simulink model "CHM2StateCtrl"  (R2018b)
settings: Solver=FixedStepDiscrete  StartTime=0.0  StopTime=10.0  FixedStep=0.01  RelTol=1e-3
undefined symbols (not defined in the file or in its folder): KeSMSuChmReqDurnTm_Val
settings Model: Creator=sn2xws  LastModifiedBy=sn2xws
settings DataIOCC: SaveFormat=StructureWithTime
settings OptimizationCC: DefaultParameterBehavior=Inlined  EnhancedBackFolding=on  PassReuseOutputArgsAs=Individual arguments  ZeroExternalMemoryAtStartup=off  ZeroInternalMemoryAtStartup=off  OptimizeBlockOrder=speed  DifferentSizesBufferReuse=on  OptimizationCustomize=off
settings DebuggingCC: ParameterTunabilityLossMsg=error
settings ModelReferenceCC: ModelReferenceNumInstancesAllowed=Single
settings SFSimCC: MATLABDynamicMemAlloc=off
settings RTWCC: SystemTargetFile=autosar.tlc  GenCodeOnly=on  TemplateMakefile=ert_default_tmf  Description=AUTOSAR  GenerateReport=on  IncludeHyperlinkInReport=on  LaunchReport=on  GenerateTraceInfo=on  GenerateTraceReport=on  GenerateTraceReportSl=on  GenerateTraceReportSf=on  GenerateTraceReportEml=on  GenerateCodeMetricsReport=on
settings CodeAppCC: ForceParamTrailComments=on  IgnoreCustomStorageClasses=off  OperatorAnnotations=on  SimulinkDataObjDesc=on  SFDataObjDesc=on  InsertBlockDesc=on
settings STFCustomTargetCC: TargetLangStandard=C99 (ISO)  MultiwordLength=256  ParMdlRefBuildCompliant=on  CompOptLevelCompliant=on  IncludeMdlTerminateFcn=off  CombineOutputUpdateFcns=on  SuppressErrorStatus=on  ERTCustomFileBanners=on  SupportNonFinite=off  SupportComplex=off  SupportContinuousTime=off  SupportNonInlinedSFcns=off  RemoveResetFunc=on  MATLABClassNameForMDSCustomization=Simulink.SoftwareTarget.ERTCustomization  AutosarCompliant=on  UseToolchainInfoCompliant=on  LookupTableObjectStructAxisOrder=2,1,3,4,...  LUTObjectStructOrderEvenSpacing=Size,Table,Breakpoints  SystemTargetFile=autosar.tlc
settings ERTTargetCC: TargetLangStandard=C99 (ISO)  ConcurrentExecutionCompliant=off  IncludeMdlTerminateFcn=off  SuppressErrorStatus=on  SupportNonFinite=off  SupportComplex=off  ModelStepFunctionPrototypeControlCompliant=off  CPPClassGenCompliant=off  AutosarCompliant=on  LookupTableObjectStructAxisOrder=2,1,3,4,...  LUTObjectStructOrderEvenSpacing=Size,Table,Breakpoints  InlinedParameterPlacement=NonHierarchical  ERTCustomFileTemplate=example_file_process.tlc  ERTFilePackagingFormat=Compact

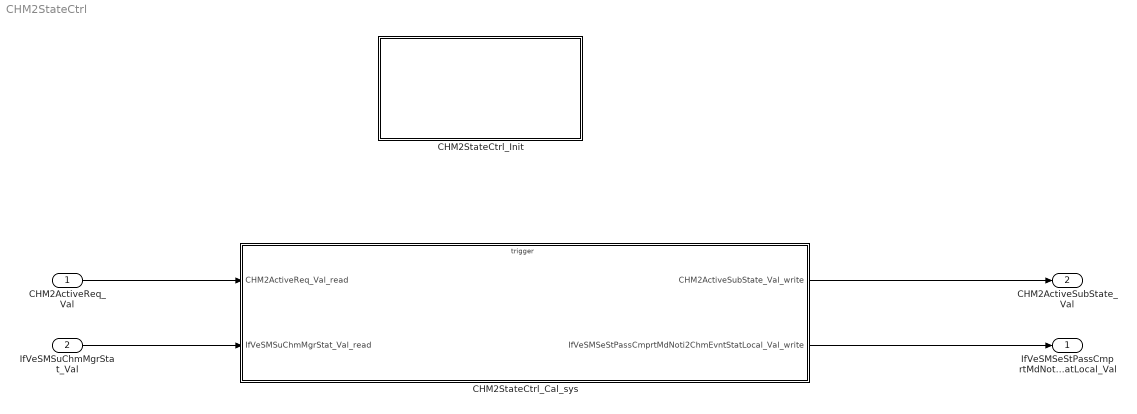
== system CHM2StateCtrl ==
  CHM2ActiveReq_Val : Inport  OutDataTypeStr=boolean  PortDimensions=1
  IfVeSMSuChmMgrStat_Val : Inport  Port=2  OutDataTypeStr=uint16  PortDimensions=1
  CHM2StateCtrl_Cal_sys : Subsystem
  CHM2StateCtrl_Init : Subsystem
  IfVeSMSeStPassCmprtMdNoti2ChmEvntStatLocal_Val : Outport  OutDataTypeStr=Enum: EventSts1  PortDimensions=1
  CHM2ActiveSubState_Val : Outport  Port=2  OutDataTypeStr=boolean  PortDimensions=1
  wires:
  CHM2ActiveReq_Val/1 -> CHM2StateCtrl_Cal_sys/1(CHM2ActiveReq_Val_read)
  IfVeSMSuChmMgrStat_Val/1 -> CHM2StateCtrl_Cal_sys/2(IfVeSMSuChmMgrStat_Val_read)
  CHM2StateCtrl_Cal_sys/1(CHM2ActiveSubState_Val_write) -> CHM2ActiveSubState_Val/1
  CHM2StateCtrl_Cal_sys/2(IfVeSMSeStPassCmprtMdNoti2ChmEvntStatLocal_Val_write) -> IfVeSMSeStPassCmprtMdNoti2ChmEvntStatLocal_Val/1

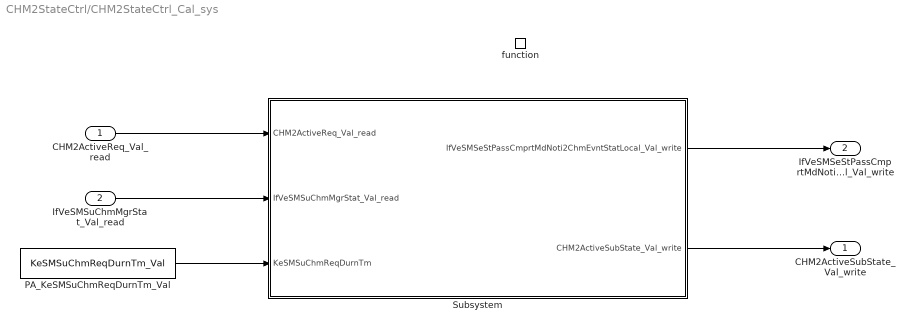
== system CHM2StateCtrl/CHM2StateCtrl_Cal_sys ==
  CHM2ActiveReq_Val_read : Inport
  IfVeSMSuChmMgrStat_Val_read : Inport  Port=2
  function : TriggerPort  TriggerType=function-call  IsSimulinkFunction=on  FunctionName=CHM2StateCtrl_Cal  VariantControl=(inherit)
  PA_KeSMSuChmReqDurnTm_Val : Constant  Value=KeSMSuChmReqDurnTm_Val
  Subsystem : Subsystem
  CHM2ActiveSubState_Val_write : Outport
      settings: EnsureOutportIsVirtual=on
  IfVeSMSeStPassCmprtMdNoti2ChmEvntStatLocal_Val_write : Outport  Port=2
      settings: EnsureOutportIsVirtual=on
  wires:
  Subsystem/2(CHM2ActiveSubState_Val_write) -> CHM2ActiveSubState_Val_write/1
  Subsystem/1(IfVeSMSeStPassCmprtMdNoti2ChmEvntStatLocal_Val_write) -> IfVeSMSeStPassCmprtMdNoti2ChmEvntStatLocal_Val_write/1
  CHM2ActiveReq_Val_read/1 -> Subsystem/1(CHM2ActiveReq_Val_read)
  IfVeSMSuChmMgrStat_Val_read/1 -> Subsystem/2(IfVeSMSuChmMgrStat_Val_read)
  PA_KeSMSuChmReqDurnTm_Val/1 -> Subsystem/3(KeSMSuChmReqDurnTm)

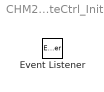
== system CHM2StateCtrl/CHM2StateCtrl_Init ==
  Event Listener : EventListener  EventName=reset

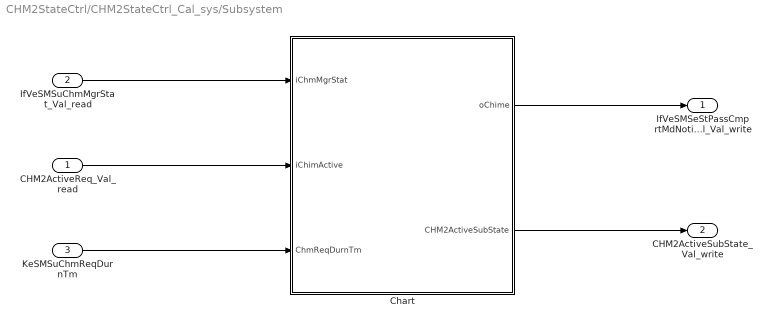
== system CHM2StateCtrl/CHM2StateCtrl_Cal_sys/Subsystem ==
  CHM2ActiveReq_Val_read : Inport
  IfVeSMSuChmMgrStat_Val_read : Inport  Port=2
  KeSMSuChmReqDurnTm : Inport  Port=3
  Chart : Stateflow chart  TreatAsAtomicUnit=on
  IfVeSMSeStPassCmprtMdNoti2ChmEvntStatLocal_Val_write : Outport
      settings: EnsureOutportIsVirtual=on
  CHM2ActiveSubState_Val_write : Outport  Port=2
      settings: EnsureOutportIsVirtual=on
  wires:
  IfVeSMSuChmMgrStat_Val_read/1 -> Chart/1(iChmMgrStat)
  CHM2ActiveReq_Val_read/1 -> Chart/2(iChimActive)
  Chart/1(oChime) -> IfVeSMSeStPassCmprtMdNoti2ChmEvntStatLocal_Val_write/1
  KeSMSuChmReqDurnTm/1 -> Chart/3(ChmReqDurnTm)
  Chart/2(CHM2ActiveSubState) -> CHM2ActiveSubState_Val_write/1

== stateflow chart CHM2StateCtrl/CHM2StateCtrl_Cal_sys/Subsystem/Chart ==
  state CHIM2Req
    en:CHM2ActiveSubState=1;
    ex:CHM2ActiveSubState=0;
  state Idle
    en:
    oChime = EventSts1.EventSts_NoAct;
  state Cancel
    en:oChime = EventSts1.EventSts_CancleChime;
  state CancelwithNoCancel
    en:oChime = EventSts1.EventSts_NoAct;
  note: $0=NO_ACTION; $1=ACTIVE; $2=CANCEL_CHIME
  (default) -> Idle
  Idle -> CHIM2Req : [iChimActive]
  Cancel -> Idle : [after(ChmReqDurnTm/10,tick)]
  CHIM2Req -> Cancel [order 1] : [!iChimActive&&iChmMgrStat==2725]
  CancelwithNoCancel -> Cancel [order 2] : [iChmMgrStat==2725]
  CancelwithNoCancel -> Idle [order 1] : [after(ChmReqDurnTm/10,tick)]
  CHIM2Req -> CancelwithNoCancel [order 2] : [!iChimActive]
  data: iChmMgrStat input; iChimActive input boolean; oChime output Enum: EventSts1; retrycnt local uint8; ChmReqDurnTm input uint8; CHM2ActiveSubState output boolean
